simulink model "mdl3"  (R2013b)
settings: Solver=ode1  StartTime=0.0  StopTime=tSim  FixedStep=h  RelTol=1e-3
values from neighbouring files (symbols this model uses):
  h = 0.0001    [test.m]
  y0 = 3    [test.m]
settings Model: Creator=JAR  LastModifiedBy=JAR

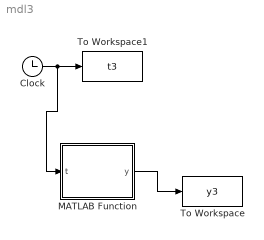
== system mdl3 ==
  Clock : Clock
  MATLAB Function : MATLAB Function  TreatAsAtomicUnit=on
  To Workspace : ToWorkspace  VariableName=y3  SampleTime=-1
  To Workspace1 : ToWorkspace  VariableName=t3  SampleTime=-1
  wires:
  Clock/1 -> MATLAB Function/1(t), To Workspace1/1
  MATLAB Function/1(y) -> To Workspace/1

== matlab function mdl3/MATLAB Function ==
  data: y0 parameter size=1; h parameter size=1; t input size=1; u parameter size=1; y output size=1
function y = fcn(y0,h,t,u)
    persistent state;
    if issempty(state)
        state = y0;
    else
        state = state + h * (-0.5 * state + u);
    end
    y = state;
end
